simulink model "control"  (R2021a)
settings: Solver=FixedStepAuto  StartTime=0.0  StopTime=10.0  RelTol=1e-3
settings Model: DataDictionary=px4_dict.sldd  Creator=DELL  LastModifiedBy=DELL
settings OptimizationCC: DefaultUnderspecifiedDataType=single

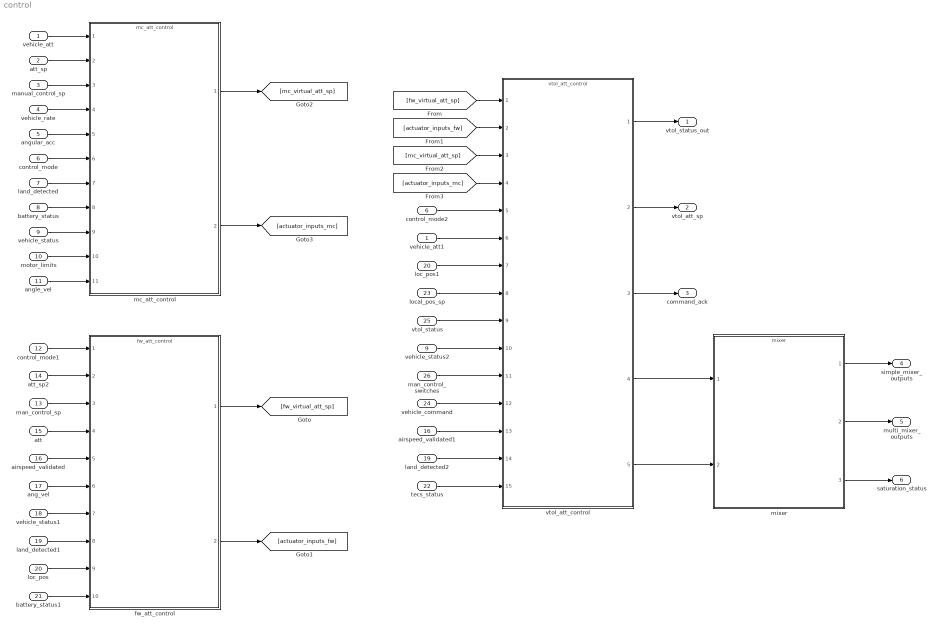
== system control ==
  vehicle_att : Inport  OutDataTypeStr=Bus: px4_vehicle_attitude  BusOutputAsStruct=on
  att_sp : Inport  Port=2  OutDataTypeStr=Bus: px4_vehicle_attitude_setpoint  BusOutputAsStruct=on
  manual_control_sp : Inport  Port=3  OutDataTypeStr=Bus: px4_manual_control_setpoint  BusOutputAsStruct=on
  vehicle_rate : Inport  Port=4  OutDataTypeStr=Bus: px4_vehicle_angular_velocity  BusOutputAsStruct=on
  angular_acc : Inport  Port=5  OutDataTypeStr=Bus: px4_vehicle_angular_acceleration  BusOutputAsStruct=on
  control_mode : Inport  Port=6  OutDataTypeStr=Bus: px4_vehicle_control_mode  BusOutputAsStruct=on
  land_detected : Inport  Port=7  OutDataTypeStr=Bus: px4_vehicle_land_detected  BusOutputAsStruct=on
  battery_status : Inport  Port=8  OutDataTypeStr=Bus: px4_battery_status  BusOutputAsStruct=on
  vehicle_status : Inport  Port=9  OutDataTypeStr=Bus: px4_vehicle_status  BusOutputAsStruct=on
  motor_limits : Inport  Port=10  OutDataTypeStr=Bus: px4_multirotor_motor_limits  BusOutputAsStruct=on
  angle_vel : Inport  Port=11  OutDataTypeStr=Bus: px4_vehicle_angular_velocity  BusOutputAsStruct=on
  control_mode1 : Inport  Port=12  OutDataTypeStr=Bus: px4_vehicle_control_mode  BusOutputAsStruct=on
  man_control_sp : Inport  Port=13  OutDataTypeStr=Bus: px4_manual_control_setpoint  BusOutputAsStruct=on
  att_sp2 : Inport  Port=14  OutDataTypeStr=Bus: px4_vehicle_attitude_setpoint  BusOutputAsStruct=on
  att : Inport  Port=15  OutDataTypeStr=Bus: px4_vehicle_attitude  BusOutputAsStruct=on
  airspeed_validated : Inport  Port=16  OutDataTypeStr=Bus: px4_airspeed_validated  BusOutputAsStruct=on
  ang_vel : Inport  Port=17  OutDataTypeStr=Bus: px4_vehicle_angular_velocity  BusOutputAsStruct=on
  vehicle_status1 : Inport  Port=18  OutDataTypeStr=Bus: px4_vehicle_status  BusOutputAsStruct=on
  land_detected1 : Inport  Port=19  OutDataTypeStr=Bus: px4_vehicle_land_detected  BusOutputAsStruct=on
  loc_pos : Inport  Port=20  OutDataTypeStr=Bus: px4_vehicle_local_position  BusOutputAsStruct=on
  battery_status1 : Inport  Port=21  OutDataTypeStr=Bus: px4_battery_status  BusOutputAsStruct=on
  tecs_status : Inport  Port=22  OutDataTypeStr=Bus: px4_tecs_status  BusOutputAsStruct=on
  local_pos_sp : Inport  Port=23  OutDataTypeStr=Bus: px4_vehicle_local_position_setpoint  BusOutputAsStruct=on
  vehicle_command : Inport  Port=24  OutDataTypeStr=Bus: px4_vehicle_command  BusOutputAsStruct=on
  vtol_status : Inport  Port=25  OutDataTypeStr=Bus: px4_vtol_vehicle_status  BusOutputAsStruct=on
  man_control_switches : Inport  Port=26  OutDataTypeStr=Bus: px4_manual_control_switches  BusOutputAsStruct=on
  airspeed_validated1 : InportShadow  Port=16  OutDataTypeStr=Bus: px4_airspeed_validated  BusOutputAsStruct=on
  control_mode2 : InportShadow  Port=6  OutDataTypeStr=Bus: px4_vehicle_control_mode  BusOutputAsStruct=on
  fw_att_control : ModelReference  ModelNameDialog=fw_att_control.slx  SimulationMode=Normal  ModelReferenceVersion=1.894
  land_detected2 : InportShadow  Port=19  OutDataTypeStr=Bus: px4_vehicle_land_detected  BusOutputAsStruct=on
  loc_pos1 : InportShadow  Port=20  OutDataTypeStr=Bus: px4_vehicle_local_position  BusOutputAsStruct=on
  mc_att_control : ModelReference  ModelNameDialog=mc_att_control.slx  SimulationMode=Normal  ModelReferenceVersion=1.1321
  mixer : ModelReference  ModelNameDialog=mixer.slx  SimulationMode=Normal  ModelReferenceVersion=1.641
  vehicle_att1 : InportShadow  OutDataTypeStr=Bus: px4_vehicle_attitude  BusOutputAsStruct=on
  vehicle_status2 : InportShadow  Port=9  OutDataTypeStr=Bus: px4_vehicle_status  BusOutputAsStruct=on
  vtol_att_control : ModelReference  ModelNameDialog=vtol_att_control.slx  SimulationMode=Normal  ModelReferenceVersion=1.1418
  vtol_status_out : Outport  OutDataTypeStr=Bus: px4_vtol_vehicle_status  BusOutputAsStruct=on
  vtol_att_sp : Outport  Port=2  OutDataTypeStr=Bus: px4_vehicle_attitude_setpoint  BusOutputAsStruct=on
  command_ack : Outport  Port=3  OutDataTypeStr=Bus: px4_vehicle_command_ack  BusOutputAsStruct=on
  simple_mixer_outputs : Outport  Port=4
  multi_mixer_outputs : Outport  Port=5
  saturation_status : Outport  Port=6
  wires:
  [actuator_inputs_mc] -> vtol_att_control/4
  mixer/1 -> simple_mixer_outputs/1
  vtol_att_control/5 -> mixer/2
  vtol_att_control/4 -> mixer/1
  [mc_virtual_att_sp] -> vtol_att_control/3
  fw_att_control/2 -> [actuator_inputs_fw]
  airspeed_validated/1 -> fw_att_control/5
  man_control_sp/1 -> fw_att_control/3
  att_sp2/1 -> fw_att_control/2
  fw_att_control/1 -> [fw_virtual_att_sp]
  [actuator_inputs_fw] -> vtol_att_control/2
  [fw_virtual_att_sp] -> vtol_att_control/1
  att/1 -> fw_att_control/4
  vtol_att_control/1 -> vtol_status_out/1
  mc_att_control/1 -> [mc_virtual_att_sp]
  mc_att_control/2 -> [actuator_inputs_mc]
  vehicle_status/1 -> mc_att_control/9
  vehicle_rate/1 -> mc_att_control/4
  man_control_switches/1 -> vtol_att_control/11
  att_sp/1 -> mc_att_control/2
  manual_control_sp/1 -> mc_att_control/3
  angular_acc/1 -> mc_att_control/5
  land_detected/1 -> mc_att_control/7
  motor_limits/1 -> mc_att_control/10
  battery_status/1 -> mc_att_control/8
  loc_pos/1 -> fw_att_control/9
  battery_status1/1 -> fw_att_control/10
  control_mode2/1 -> vtol_att_control/5
  angle_vel/1 -> mc_att_control/11
  vtol_att_control/2 -> vtol_att_sp/1
  vtol_att_control/3 -> command_ack/1
  loc_pos1/1 -> vtol_att_control/7
  vehicle_status1/1 -> fw_att_control/7
  vtol_status/1 -> vtol_att_control/9
  local_pos_sp/1 -> vtol_att_control/8
  vehicle_att/1 -> mc_att_control/1
  mixer/2 -> multi_mixer_outputs/1
  mixer/3 -> saturation_status/1
  vehicle_status2/1 -> vtol_att_control/10
  vehicle_command/1 -> vtol_att_control/12
  control_mode/1 -> mc_att_control/6
  vehicle_att1/1 -> vtol_att_control/6
  land_detected2/1 -> vtol_att_control/14
  airspeed_validated1/1 -> vtol_att_control/13
  ang_vel/1 -> fw_att_control/6
  control_mode1/1 -> fw_att_control/1
  land_detected1/1 -> fw_att_control/8
  tecs_status/1 -> vtol_att_control/15
